simulink model "Delay5"  (R2017b)
settings: Solver=FixedStepDiscrete  StartTime=0.0  StopTime=10.0  FixedStep=0.200000  RelTol=1e-3  EnableMultiTasking=on
settings Model: Creator=hbourbou  LastModifiedBy=hbourbou
settings DataIOCC: LimitDataPoints=on  SaveFormat=Structure
settings OptimizationCC: LifeSpan=inf
settings DebuggingCC: SFUnexpectedBacktrackingDiag=warning  SFNoUnconditionalDefaultTransitionDiag=warning  SFExecutionAtInitializationDiag=none
settings HardwareCC: ProdBitPerPointer=32  ProdBitPerSizeT=32  ProdBitPerPtrDiffT=32  ProdLargestAtomicFloat=None  ProdIntDivRoundTo=Undefined  ProdEndianess=Unspecified  ProdWordSize=32  ProdHWDeviceType=32-bit Generic
settings ModelReferenceCC: PropagateSignalLabelsOutOfModel=off
settings CodeAppCC: StateflowObjectComments=on
settings GRTTargetCC: TargetLangStandard=C89/C90 (ANSI)  GeneratePreprocessorConditionals=Disable all
settings ConfigComp: CovMetricSettings=dw  CovHtmlReporting=on  CovSaveCumulativeToWorkspaceVar=on  CovSaveSingleToWorkspaceVar=on  CovExternalEMLEnable=off

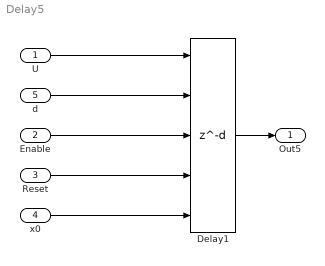
== system Delay5 ==
  U : Inport  PortDimensions=2
  Enable : Inport  Port=2  PortDimensions=1
  Reset : Inport  Port=3  OutDataTypeStr=boolean  PortDimensions=1
  x0 : Inport  Port=4
  d : Inport  Port=5
  Delay1 : Delay  DelayLengthSource=Input port  InitialConditionSource=Input port  ExternalReset=Falling  ShowEnablePort=on
      settings: InputPortMap=u0,p1,e6,r5,p4
  Out5 : Outport
  wires:
  Enable/1 -> Delay1/3
  Reset/1 -> Delay1/4
  x0/1 -> Delay1/5
  U/1 -> Delay1/1
  d/1 -> Delay1/2
  Delay1/1 -> Out5/1
